simulink model "DC_Motor_Model"  (R2025b)
settings: Solver=ode15s  StartTime=0.0  StopTime=5  RelTol=1e-3
values from neighbouring files (symbols this model uses):
  B = 0.1    [motor_parameters.m]
  J = 0.01    [motor_parameters.m]
  Ke = 0.01    [motor_parameters.m]
  Kt = 0.01    [motor_parameters.m]
  L = 0.5    [motor_parameters.m]
  R = 1    [motor_parameters.m]
  TL = 0.1    [motor_parameters.m]
libraries: slpidlib x1
settings Model: Creator=KEVIN  LastModifiedBy=KEVIN

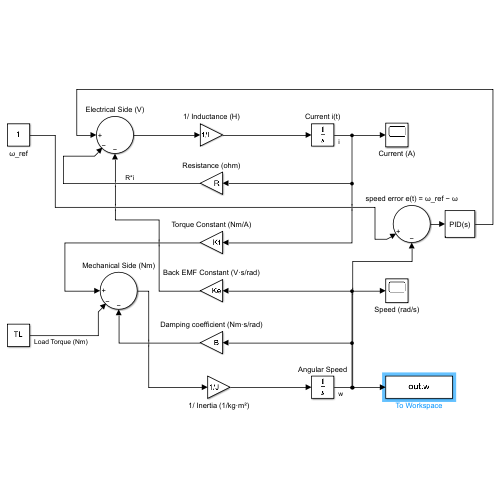
[thumbnail: Simulink's stored preview of the top-level diagram]
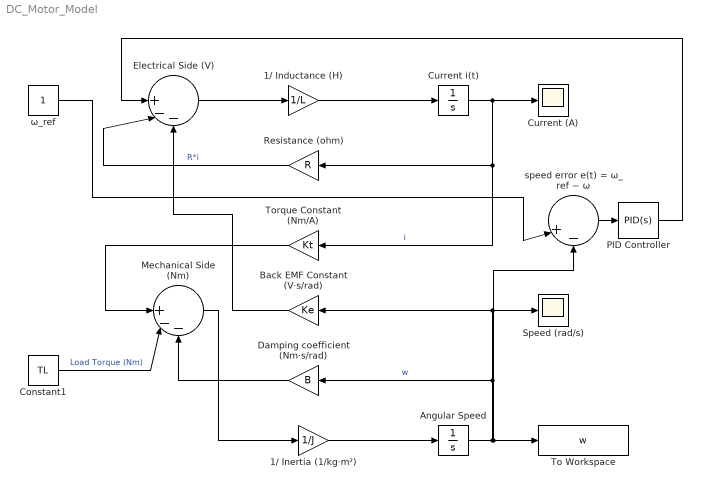
== system DC_Motor_Model ==
  1/ Inductance (H) : Gain  Gain=1/L
  1/ Inertia (1/kg·m²) : Gain  Gain=1/J
  Angular Speed : Integrator
  Back EMF Constant (V·s/rad) : Gain  Gain=Ke
  Constant1 : Constant  Value=TL
  Current (A) : Scope
      settings: ActiveDisplayYMinimum=-1  ActiveDisplayYMaximum=1
  Current i(t) : Integrator
  Damping coefficient (Nm·s/rad) : Gain  Gain=B
  Electrical Side (V) : Sum  Inputs=||||+|-|-
  Mechanical Side (Nm) : Sum  Inputs=||||+|-|-
  PID Controller : slpidlib/PID Controller  Controller=PID  Form=Parallel  TimeDomain=Continuous-time  UseExternalTs=off  SampleTime=-1  IntegratorMethod=Forward Euler  FilterMethod=Forward Euler  ControllerParametersSource=internal  P=5  I=12  UseKiTs=off  D=0.2  UseExternalDerivativeSource=off  N=100  UseFilter=on  TunerSelectOption=Transfer Function Based (PID Tuner App)  InitialConditionSource=internal  InitialConditionForIntegrator=0  InitialConditionForFilter=0  DifferentiatorICPrevScaledInput=0  ExternalReset=none  TrackingMode=off  Kt=1  LimitOutput=off  SatLimitsSource=internal  UpperSaturationLimit=inf  LowerSaturationLimit=-inf  LinearizeAsGain=on  AntiWindupMode=none  Kb=1  LimitIntegrator=off  UpperIntegratorSaturationLimit=inf  LowerIntegratorSaturationLimit=-inf  POutMin=[]  POutMax=[]  IOutMin=[]  IOutMax=[]  DOutMin=[]  DOutMax=[]  NOutMin=[]  NOutMax=[]  SumOutMin=[]  SumOutMax=[]  SaturationOutMin=[]  SaturationOutMax=[]  PParamMin=[]  PParamMax=[]  IParamMin=[]  IParamMax=[]  DParamMin=[]  DParamMax=[]  NParamMin=[]  NParamMax=[]  KbParamMin=[]  KbParamMax=[]  KtParamMin=[]  KtParamMax=[]  KbOutMin=[]  KbOutMax=[]  KtOutMin=[]  KtOutMax=[]  IntegratorOutMin=[]  IntegratorOutMax=[]  FilterOutMin=[]  FilterOutMax=[]  SumI1OutMin=[]  SumI1OutMax=[]  SumI2OutMin=[]  SumI2OutMax=[]  SumI3OutMin=[]  SumI3OutMax=[]  SumI4OutMin=[]  SumI4OutMax=[]  SumDOutMin=[]  SumDOutMax=[]  DifferentiatorOutMin=[]  DifferentiatorOutMax=[]  FilterDiffOutCoefMin=[]  FilterDiffOutCoefMax=[]  ReciprocalOutMin=[]  ReciprocalOutMax=[]  SumDenOutMin=[]  SumDenOutMax=[]  SumNumOutMin=[]  SumNumOutMax=[]  DivideOutMin=[]  DivideOutMax=[]  UdiffTsProdOutMin=[]  UdiffTsProdOutMax=[]  NTsProdOutMin=[]  NTsProdOutMax=[]  UintegralTsProdOutMin=[]  UintegralTsProdOutMax=[]  UngainTsProdOutMin=[]  UngainTsProdOutMax=[]  ClampingZeroOutDataTypeStr=Inherit: Inherit via back propagation  ClampingZeroOutMin=[]  ClampingZeroOutMax=[]  FilterDenConstantOutDataTypeStr=Inherit: Inherit via back propagation  FilterDenConstantOutMin=[]  FilterDenConstantOutMax=[]  PCopyOutDataTypeStr=Inherit: Inherit via back propagation  PCopyOutMin=[]  PCopyOutMax=[]  NCopyOutDataTypeStr=Inherit: Inherit via back propagation  NCopyOutMin=[]  NCopyOutMax=[]  IntegratorContinuousStateAttributes=''  IntegratorStateMustResolveToSignalObject=off  IntegratorRTWStateStorageClass=Auto  FilterContinuousStateAttributes=''  FilterStateMustResolveToSignalObject=off  FilterRTWStateStorageClass=Auto  ParallelPVariant=InternalParameters  IdealPVariant=Disabled  IVariant=InternalParameters  DVariant=InternalParameters  IntegratorVariant=Continuous  SatVariant=Disabled  AWVariant=Passthrough  PCopyVariant=Disabled  TRVariant=Disabled  FdbkBlocksVariant=Forward  IdealPFdbkVariant=Disabled  SatFdbkVariant=Disabled  DerivativeFilterVariant=ContFilter  NVariant=InternalParameters  NCopyVariant=Disabled  FilterICVariant=InternalICsFilter  IntegratorICVariant=InternalICs  ExternalResetVariant=Disabled  TRSumVariant=Passthrough  SumFdbkVariant=Disabled  SumVariant=Sum_PID  TsampFilterVariant=InternalTs  TsampNgainVariant=Passthrough  TsampIntegralVariant=Disabled_SignalSpec  ExternalSaturationOutDataTypeStr=Inherit: Same as second input  DerivativeSourceVariant=ErrorSignal  PreIntVariant=InternalPreInt
  Resistance (ohm) : Gain  Gain=R
  Speed (rad/s) : Scope
      settings: ActiveDisplayYMinimum=-0.86237101270360073  ActiveDisplayYMaximum=1.1922841499396222
  To Workspace : ToWorkspace  VariableName=w  SaveFormat=Structure With Time  SampleTime=-1
  Torque Constant (Nm/A) : Gain  Gain=Kt
  speed error e(t) = ω_ref − ω : Sum  Inputs=||||+|-
  ω_ref : Constant
  wires:
  Electrical Side (V)/1 -> 1/ Inductance (H)/1
  1/ Inductance (H)/1 -> Current i(t)/1
  ω_ref/1 -> speed error e(t) = ω_ref − ω/1
  Current i(t)/1 -> Current (A)/1, Torque Constant (Nm/A)/1, Resistance (ohm)/1  "i"
  Resistance (ohm)/1 -> Electrical Side (V)/2  "R*i"
  Back EMF Constant (V·s/rad)/1 -> Electrical Side (V)/3
  Angular Speed/1 -> To Workspace/1, speed error e(t) = ω_ref − ω/2, Speed (rad/s)/1, Back EMF Constant (V·s/rad)/1, Damping coefficient (Nm·s/rad)/1  "w"
  Constant1/1 -> Mechanical Side (Nm)/2  "Load Torque (Nm)"
  Torque Constant (Nm/A)/1 -> Mechanical Side (Nm)/1
  Damping coefficient (Nm·s/rad)/1 -> Mechanical Side (Nm)/3
  Mechanical Side (Nm)/1 -> 1/ Inertia (1/kg·m²)/1
  1/ Inertia (1/kg·m²)/1 -> Angular Speed/1
  speed error e(t) = ω_ref − ω/1 -> PID Controller/1
  PID Controller/1 -> Electrical Side (V)/1
